simulink model "uklad1"  (R2021a)
settings: Solver=VariableStepAuto  StartTime=0.0  StopTime=10.0  RelTol=1e-3
settings Model: Creator=ADMIN  LastModifiedBy=ADMIN

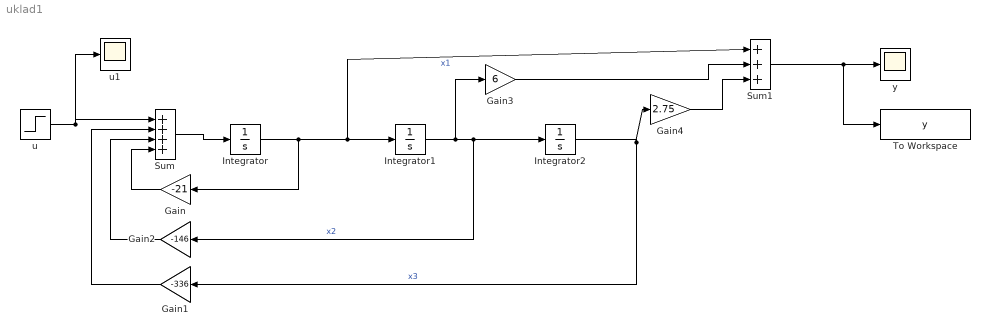
== system uklad1 ==
  Gain : Gain  Gain=-21
  Gain1 : Gain  Gain=-336
  Gain2 : Gain  Gain=-146
  Gain3 : Gain  Gain=6
  Gain4 : Gain  Gain=2.75
  Integrator : Integrator  InitialCondition=1
  Integrator1 : Integrator  InitialCondition=-1
  Integrator2 : Integrator  InitialCondition=1
  Sum : Sum  Inputs=|++++
  Sum1 : Sum  Inputs=|+++
  To Workspace : ToWorkspace  VariableName=y  SaveFormat=Structure With Time  SampleTime=-1
  u : Step  SampleTime=0
  u1 : Scope
  y : Scope
  wires:
  Sum/1 -> Integrator/1
  Gain/1 -> Sum/4
  Integrator/1 -> Sum1/1, Integrator1/1, Gain/1  "x1"
  Integrator1/1 -> Gain3/1, Gain2/1, Integrator2/1  "x2"
  Integrator2/1 -> Gain4/1, Gain1/1  "x3"
  Gain1/1 -> Sum/2
  Gain2/1 -> Sum/3
  Gain4/1 -> Sum1/3
  Gain3/1 -> Sum1/2
  u/1 -> u1/1, Sum/1
  Sum1/1 -> To Workspace/1, y/1
